simulink subsystem "TX"  (R2022b)
settings: Solver=VariableStepAuto  StartTime=0.0  StopTime=10.0  RelTol=1e-3
settings Model: Creator=Ali-Laptop  LastModifiedBy=Ali-Laptop

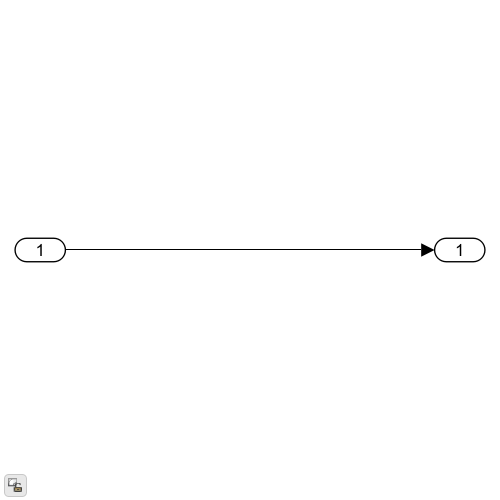
[thumbnail: Simulink's stored preview of the top-level diagram]
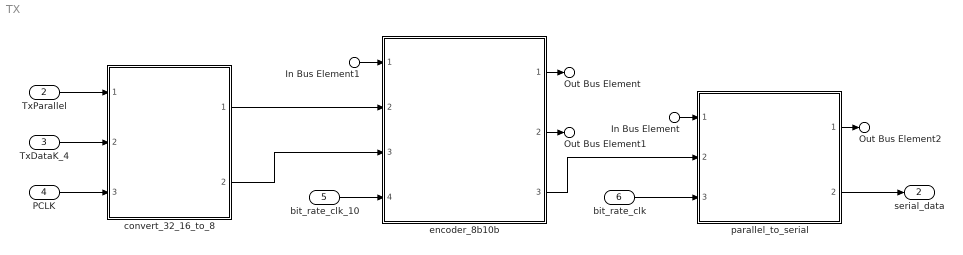
== system TX ==
  In Bus Element : Inport  PortName=digital_out  Element=Serial_out
  In Bus Element1 : Inport  PortName=digital_out  Element=TxParallel_10_out
  TxParallel : Inport  Port=2
  TxDataK_4 : Inport  Port=3
  PCLK : Inport  Port=4
  bit_rate_clk_10 : Inport  Port=5
  bit_rate_clk : Inport  Port=6
  convert_32_16_to_8 : Subsystem  ReferencedSubsystem=convert_32_16_to_8
  encoder_8b10b : Subsystem  ReferencedSubsystem=encoder_8b10b
  parallel_to_serial : Subsystem  ReferencedSubsystem=parallel_to_serial
  Out Bus Element : Outport  PortName=digital_in  Element=TxDataK_in
  Out Bus Element1 : Outport  PortName=digital_in  Element=TxParallel_8_in
  Out Bus Element2 : Outport  PortName=digital_in  Element=TxParallel_10_in
  serial_data : Outport  Port=2
  wires:
  TxParallel/1 -> convert_32_16_to_8/1
  encoder_8b10b/1 -> Out Bus Element/1
  encoder_8b10b/2 -> Out Bus Element1/1
  convert_32_16_to_8/2 -> encoder_8b10b/3
  In Bus Element1/1 -> encoder_8b10b/1
  In Bus Element/1 -> parallel_to_serial/1
  parallel_to_serial/1 -> Out Bus Element2/1
  parallel_to_serial/2 -> serial_data/1
  TxDataK_4/1 -> convert_32_16_to_8/2
  convert_32_16_to_8/1 -> encoder_8b10b/2
  encoder_8b10b/3 -> parallel_to_serial/2
  bit_rate_clk_10/1 -> encoder_8b10b/4
  bit_rate_clk/1 -> parallel_to_serial/3
  PCLK/1 -> convert_32_16_to_8/3
